simulink model "cvac_if_controller"  (R2026a)
settings: Solver=FixedStepDiscrete  StopTime=2  FixedStep=cvac.TsFast
values from neighbouring files (symbols this model uses):
  cvac = struct    [cvac_if_model_init.m]
settings Model: Creator=ASUS  LastModifiedBy=ASUS

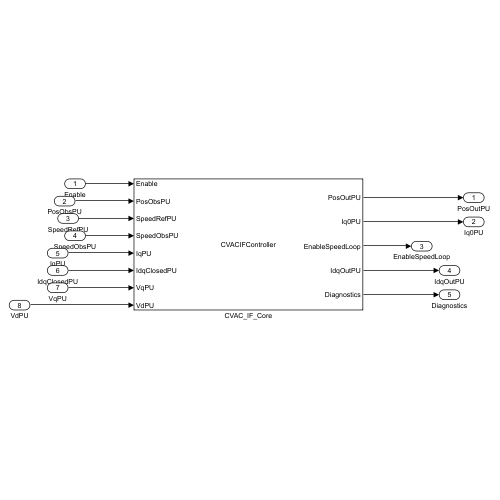
[thumbnail: Simulink's stored preview of the top-level diagram]
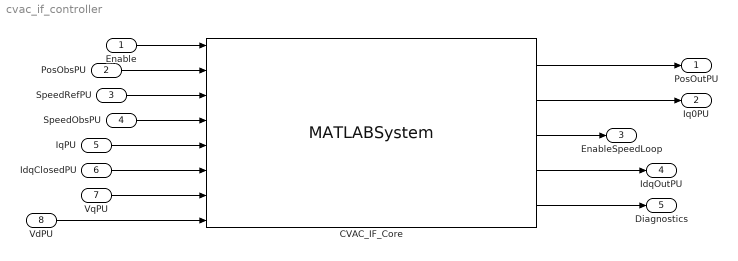
== system cvac_if_controller ==
  Enable : Inport  OutDataTypeStr=boolean  SampleTime=cvac.TsFast
  PosObsPU : Inport  Port=2  OutDataTypeStr=single  SampleTime=cvac.TsFast
  SpeedRefPU : Inport  Port=3  OutDataTypeStr=single  SampleTime=cvac.TsFast
  SpeedObsPU : Inport  Port=4  OutDataTypeStr=single  SampleTime=cvac.TsFast
  IqPU : Inport  Port=5  OutDataTypeStr=single  SampleTime=cvac.TsFast
  IdqClosedPU : Inport  Port=6  OutDataTypeStr=single  PortDimensions=2  SampleTime=cvac.TsFast
  VqPU : Inport  Port=7  OutDataTypeStr=single  SampleTime=cvac.TsFast
  VdPU : Inport  Port=8  OutDataTypeStr=single  SampleTime=cvac.TsFast
  CVAC_IF_Core : MATLABSystem  System=CVACIFController  TsFast=cvac.TsFast  TsSlow=cvac.TsSlow  PolePairs=cvac.PolePairs  SpeedBaseRpm=cvac.SpeedBaseRpm  CurrentBaseA=cvac.CurrentBaseA  VoltageBaseV=cvac.VoltageBaseV  LqH=cvac.LqH  FluxWb=cvac.FluxWb  IStartA=cvac.IStartA  IAlignA=cvac.IAlignA  IMinA=cvac.IMinA  OmegaRefRadps=cvac.OmegaRefRadps  OmegaThetaOnRadps=cvac.OmegaThetaOnRadps  BetaSeedRadps2=cvac.BetaSeedRadps2  BetaMaxRadps2=cvac.BetaMaxRadps2  DeltaOmegaMaxRadps=cvac.DeltaOmegaMaxRadps  Ktheta=cvac.Ktheta  Kdp=cvac.Kdp  TorqueMinNm=cvac.TorqueMinNm  HpfCutoffHz=cvac.HpfCutoffHz  KpBeta=cvac.KpBeta  KiBeta=cvac.KiBeta  KawBeta=cvac.KawBeta  KpCurrent=cvac.KpCurrent  KiCurrent=cvac.KiCurrent  KawCurrent=cvac.KawCurrent  CurrentRiseAps=cvac.CurrentRiseAps  CurrentFallAps=cvac.CurrentFallAps  AlignTimeS=cvac.AlignTimeS  VectorRotateTimeS=cvac.VectorRotateTimeS  ThetaValidTimeS=cvac.ThetaValidTimeS  ConstSpeedMinTimeS=cvac.ConstSpeedMinTimeS  HandoffQualifyTimeS=cvac.HandoffQualifyTimeS  StartupTimeoutS=cvac.StartupTimeoutS  ThetaEstimateLimitRad=cvac.ThetaEstimateLimitRad  ThetaFaultLimitRad=cvac.ThetaFaultLimitRad  ConstSpeedAngleLimitRad=cvac.ConstSpeedAngleLimitRad  HandoffAngleLimitRad=cvac.HandoffAngleLimitRad  HandoffSpeedLimitPU=cvac.HandoffSpeedLimitPU  HandoffUnderspeedLimitPU=cvac.HandoffUnderspeedLimitPU  CurrentTrackingLimitA=cvac.CurrentTrackingLimitA  CurrentTrackingTimeS=cvac.CurrentTrackingTimeS  VoltageSaturationPU=cvac.VoltageSaturationPU  VoltageSaturationTimeS=cvac.VoltageSaturationTimeS  SimulateUsing=Interpreted execution
      mask Type: CVACIFController
  PosOutPU : Outport
  Iq0PU : Outport  Port=2
  EnableSpeedLoop : Outport  Port=3
  IdqOutPU : Outport  Port=4
  Diagnostics : Outport  Port=5
  wires:
  Enable/1 -> CVAC_IF_Core/1
  PosObsPU/1 -> CVAC_IF_Core/2
  SpeedRefPU/1 -> CVAC_IF_Core/3
  SpeedObsPU/1 -> CVAC_IF_Core/4
  IqPU/1 -> CVAC_IF_Core/5
  IdqClosedPU/1 -> CVAC_IF_Core/6
  VqPU/1 -> CVAC_IF_Core/7
  VdPU/1 -> CVAC_IF_Core/8
  CVAC_IF_Core/1 -> PosOutPU/1
  CVAC_IF_Core/2 -> Iq0PU/1
  CVAC_IF_Core/3 -> EnableSpeedLoop/1
  CVAC_IF_Core/4 -> IdqOutPU/1
  CVAC_IF_Core/5 -> Diagnostics/1
